simulink library "INT_CrCtl_StTrans"  (R2016b)
settings: Solver=VariableStepAuto  StartTime=0.0  StopTime=10.0  RelTol=1e-3
settings Model: Creator=guanxiaoxing  LastModifiedBy=guanxiaoxing

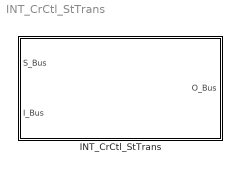
== system INT_CrCtl_StTrans ==
  INT_CrCtl_StTrans : Subsystem

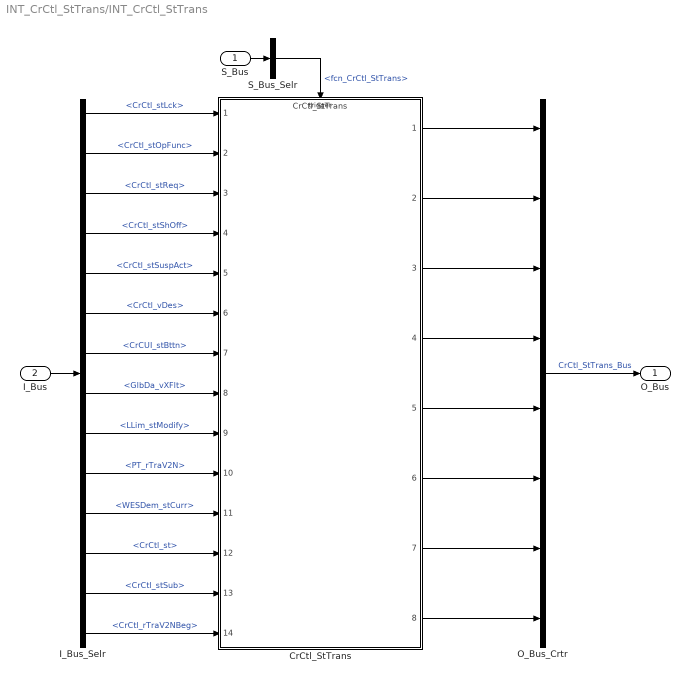
== system INT_CrCtl_StTrans/INT_CrCtl_StTrans ==
  S_Bus : Inport
  I_Bus : Inport  Port=2
  CrCtl_StTrans : ModelReference  ModelNameDialog=CrCtl_StTrans  SimulationMode=Normal  ModelReferenceVersion=1.55  TriggerPortName=function  TriggerPortTriggerType=function-call  TriggerPortStatesWhenEnabling=held
  I_Bus_Selr : BusSelector  OutputSignals=CrCtl_stLck,CrCtl_stOpFunc,CrCtl_stReq,CrCtl_stShOff,CrCtl_stSuspAct,CrCtl_vDes,CrCUI_stBttn,GlbDa_vXFlt,LLim_stModify,PT_rTraV2N,WESDem_stCurr,CrCtl_st,CrCtl_stSub,CrCtl_rTraV2NBeg
  O_Bus_Crtr : BusCreator  Inputs=8
  S_Bus_Selr : BusSelector  OutputSignals=fcn_CrCtl_StTrans
  O_Bus : Outport
  wires:
  S_Bus_Selr/1 -> CrCtl_StTrans/Trigger  "<fcn_CrCtl_StTrans>"
  S_Bus/1 -> S_Bus_Selr/1
  I_Bus/1 -> I_Bus_Selr/1
  I_Bus_Selr/1 -> CrCtl_StTrans/1  "<CrCtl_stLck>"
  I_Bus_Selr/2 -> CrCtl_StTrans/2  "<CrCtl_stOpFunc>"
  I_Bus_Selr/3 -> CrCtl_StTrans/3  "<CrCtl_stReq>"
  I_Bus_Selr/4 -> CrCtl_StTrans/4  "<CrCtl_stShOff>"
  I_Bus_Selr/5 -> CrCtl_StTrans/5  "<CrCtl_stSuspAct>"
  I_Bus_Selr/6 -> CrCtl_StTrans/6  "<CrCtl_vDes>"
  I_Bus_Selr/7 -> CrCtl_StTrans/7  "<CrCUI_stBttn>"
  I_Bus_Selr/8 -> CrCtl_StTrans/8  "<GlbDa_vXFlt>"
  I_Bus_Selr/9 -> CrCtl_StTrans/9  "<LLim_stModify>"
  I_Bus_Selr/10 -> CrCtl_StTrans/10  "<PT_rTraV2N>"
  I_Bus_Selr/11 -> CrCtl_StTrans/11  "<WESDem_stCurr>"
  I_Bus_Selr/12 -> CrCtl_StTrans/12  "<CrCtl_st>"
  I_Bus_Selr/13 -> CrCtl_StTrans/13  "<CrCtl_stSub>"
  I_Bus_Selr/14 -> CrCtl_StTrans/14  "<CrCtl_rTraV2NBeg>"
  O_Bus_Crtr/1 -> O_Bus/1  "CrCtl_StTrans_Bus"
  CrCtl_StTrans/1 -> O_Bus_Crtr/1
  CrCtl_StTrans/2 -> O_Bus_Crtr/2
  CrCtl_StTrans/3 -> O_Bus_Crtr/3
  CrCtl_StTrans/4 -> O_Bus_Crtr/4
  CrCtl_StTrans/5 -> O_Bus_Crtr/5
  CrCtl_StTrans/6 -> O_Bus_Crtr/6
  CrCtl_StTrans/7 -> O_Bus_Crtr/7
  CrCtl_StTrans/8 -> O_Bus_Crtr/8
